simulink model "sistema_completo_despues_coloquio"  (R2023a)
settings: Solver=VariableStepAuto  StartTime=0  StopTime=15  FixedStep=1e-6  MaxStep=1e-3  RelTol=1e-3
values from neighbouring files (symbols this model uses):
  alpha_Cu = 3.9e-3    (= 0.0039)    [variables.m]
  b_a = J_eq * (2*zeta + 1) * omega_pos    [Polos_con_Jeq.m]
  b_eq = b_eq_max    [FrecuenciaNatural_Amortiguamiento.m]    (also in variables.m = 2.19444444444e-05)
  C_ts = 0.818    [variables.m]
  J_eq = J_eq_max    [FrecuenciaNatural_Amortiguamiento.m]    (also in variables.m = 4.58263888889e-05)
  k_l = m*l_cm + m_l*l_l    (= 1)    [variables.m]
  K_sa = J_eq * (2*zeta + 1) * omega_pos^2    [Polos_con_Jeq.m]
  K_sia = J_eq * omega_pos^3    [Polos_con_Jeq.m]
  L_d = 6.6e-3    (= 0.0066)    [variables.m]
  L_ls = 0.8e-3    (= 0.0008)    [variables.m]
  L_q = 5.8e-3    (= 0.0058)    [variables.m]
  lambda_m = 0.016    [variables.m]
  Pp = 3    [variables.m]
  r = 120    [esp_de_operacion.m]    (also in variables.m)
  R_ts = 146.7    [variables.m]
  T_s_ref = 20    [Polos_ceros_Rs.m]
undefined symbols (not defined in the file or in its folder): k_i, k_omega2, k_theta2, omega_n_i, omega_n_pos, omega_n_v, R_s_ref, tau, Vsl_max, zitta
libraries: SignalEditorBlockLib x5
settings Model: Creator=juanf  LastModifiedBy=Juan
settings DataIOCC: Refine=8

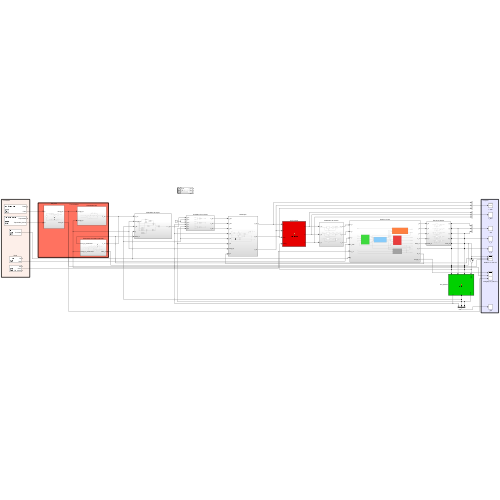
[thumbnail: Simulink's stored preview of the top-level diagram]
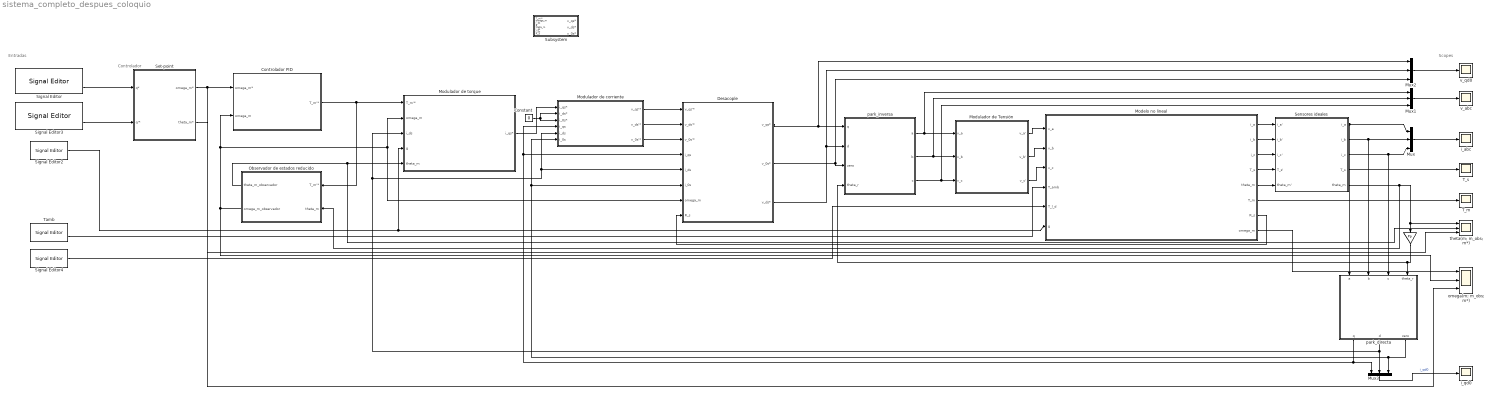
== system sistema_completo_despues_coloquio ==
  note: Controlador
  note: Scopes
  note: Entradas
  " " : Gain  Gain=Pp
  Constant : Constant  Value=0
  Controlador PID : Subsystem
  Desacople : Subsystem
  Modelo no lineal : Subsystem
  Modulador de Tensión : Subsystem
  Modulador de corriente : Subsystem
  Modulador de torque : Subsystem
  Mux{,1..3} (4 alike) : Mux  Inputs=3
  Observador de estados reducido : Subsystem
  Sensores ideales : Subsystem
  Set-point : Subsystem
  Signal Editor : SignalEditorBlockLib/Signal Editor  FileName=Consigna_Theta.mat  ActiveScenario=ConsignaTheta  ActiveSignal=Theta  IsBus=off  OutputBusObjectStr=Bus: BusObject  SampleTime=0  ZeroCross=off  OutputAfterFinalValue=Setting to zero  Unit=inherit  PreserveSignalName=on  ApplySigPropsToAllScenarios=on
  Signal Editor2 : SignalEditorBlockLib/Signal Editor  FileName=D:\Facultad\AyME\Automatica-y-maquinas-electricas-final\Matlab - Simulink\señales\g.mat  ActiveScenario=g  ActiveSignal=Constant  IsBus=off  OutputBusObjectStr=Bus: BusObject  SampleTime=0  Interpolate=off  ZeroCross=off  OutputAfterFinalValue=Setting to zero  Unit=inherit  PreserveSignalName=on  ApplySigPropsToAllScenarios=on
  Signal Editor3 : SignalEditorBlockLib/Signal Editor  FileName=D:\Facultad\AyME\Automatica-y-maquinas-electricas-final\Matlab - Simulink\señales\señal_omega_suave.mat  ActiveScenario=ConsignaOmega  ActiveSignal=Trapezoidal  IsBus=off  OutputBusObjectStr=Bus: BusObject  SampleTime=0  Interpolate=off  ZeroCross=off  OutputAfterFinalValue=Setting to zero  Unit=inherit  PreserveSignalName=on  ApplySigPropsToAllScenarios=on
  Signal Editor4 : SignalEditorBlockLib/Signal Editor  FileName=D:\Facultad\AyME\Automatica-y-maquinas-electricas-final\Matlab - Simulink\señales\Tld_15s.mat  ActiveScenario=Tld  ActiveSignal=Tld  IsBus=off  OutputBusObjectStr=Bus: BusObject  SampleTime=0  Interpolate=off  ZeroCross=off  OutputAfterFinalValue=Setting to zero  Unit=inherit  PreserveSignalName=on  ApplySigPropsToAllScenarios=on
  Subsystem : Subsystem
  T_m : Scope
  T_s : Scope
  Tamb : SignalEditorBlockLib/Signal Editor  FileName=D:\Facultad\AyME\Automatica-y-maquinas-electricas-final\Matlab - Simulink\señales\senal_Tamb.mat  ActiveScenario=T_amb  ActiveSignal=T0  IsBus=off  OutputBusObjectStr=Bus: BusObject  SampleTime=0  Interpolate=off  ZeroCross=off  OutputAfterFinalValue=Setting to zero  Unit=inherit  PreserveSignalName=on  ApplySigPropsToAllScenarios=on
  i_abc : Scope
  i_qd0 : Scope
  omega(m; m_obs; m*) : Scope  NumInputPorts=3
  park_directa : MATLAB Function  TreatAsAtomicUnit=on
  park_inversa : MATLAB Function  TreatAsAtomicUnit=on
  theta(m; m_obs; m*) : Scope  NumInputPorts=3
  v_abc : Scope
  v_qd0 : Scope
  wires:
  park_inversa/1(a) -> Mux1/1, Modulador de Tensión/1(v_a)
  park_inversa/2(b) -> Mux1/2, Modulador de Tensión/2(v_b)
  park_inversa/3(c) -> Mux1/3, Modulador de Tensión/3(v_c)
  Modulador de Tensión/1(v_a') -> Modelo no lineal/1(v_a)
  Modulador de Tensión/2(v_b') -> Modelo no lineal/2(v_b)
  Modulador de Tensión/3(v_c') -> Modelo no lineal/3(v_c)
  Modelo no lineal/1(i_a) -> Sensores ideales/1(i_a')
  Modelo no lineal/2(i_b) -> Sensores ideales/2(i_b')
  Modelo no lineal/3(i_c) -> Sensores ideales/3(i_c')
  Modelo no lineal/4(T_s) -> Sensores ideales/4(T_s')
  Modelo no lineal/5(theta_m) -> Sensores ideales/5(theta_m')
  Modelo no lineal/6(T_m) -> T_m/1
  Sensores ideales/1(i_a) -> Mux/1, park_directa/1(a)
  Sensores ideales/2(i_b) -> Mux/2, park_directa/2(b)
  Sensores ideales/3(i_c) -> Mux/3, park_directa/3(c)
  Modelo no lineal/8(omega_m) -> omega(m; m_obs; m*)/1
  Desacople/1(v_qs*) -> Mux2/1, park_inversa/1(q)
  Sensores ideales/4(T_s) -> T_s/1
  park_directa/1(q) -> Modulador de corriente/4(i_qs), Desacople/4(i_qs), Mux3/1
  park_directa/2(d) -> Mux3/2, Modulador de torque/3(i_ds), Modulador de corriente/5(i_ds), Desacople/5(i_ds)
  park_directa/3(zero) -> Mux3/3, Modulador de corriente/6(i_0s), Desacople/6(i_0s)
  Sensores ideales/5(theta_m) -> " "/1, theta(m; m_obs; m*)/1, Observador de estados reducido/2(theta_m)
  " "/1 -> park_inversa/4(theta_r), park_directa/4(theta_r)
  Mux/1 -> i_abc/1
  Mux1/1 -> v_abc/1
  Mux2/1 -> v_qd0/1
  Mux3/1 -> i_qd0/1  "i_qd0"
  Desacople/3(v_ds*) -> Mux2/2, park_inversa/2(d)
  Signal Editor2/1 -> Modulador de torque/4(g), Modelo no lineal/6(g)
  Observador de estados reducido/2(omega_m_observador) -> omega(m; m_obs; m*)/2, Controlador PID/2(omega_m), Modulador de torque/2(omega_m), Desacople/7(omega_m)
  Modulador de corriente/1(v_qs'*) -> Desacople/1(v_qs'*)
  Modulador de corriente/2(v_ds'*) -> Desacople/2(v_ds'*)
  Modulador de corriente/3(v_0s'*) -> Desacople/3(v_0s'*)
  Constant/1 -> Modulador de corriente/2(i_ds*), Modulador de corriente/3(i_0s*)
  Set-point/1(omega_m*) -> Controlador PID/1(omega_m*), omega(m; m_obs; m*)/3
  Tamb/2 -> Modelo no lineal/4(T_amb)
  Modulador de torque/1(i_qs*) -> Modulador de corriente/1(i_qs*)
  Controlador PID/1(T_m'*) -> Observador de estados reducido/1(T_m'*), Modulador de torque/1(T_m'*)
  Observador de estados reducido/1(theta_m_observador) -> theta(m; m_obs; m*)/2, Modulador de torque/5(theta_m)
  Desacople/2(v_0s*) -> park_inversa/3(zero), Mux2/3
  Modelo no lineal/7(R_s) -> Desacople/8(R_s)
  Set-point/2(theta_m*) -> theta(m; m_obs; m*)/3
  Signal Editor4/2 -> Modelo no lineal/5(T_l_d)
  Signal Editor/2 -> Set-point/1(q*)
  Signal Editor3/2 -> Set-point/2(q'*)

== system sistema_completo_despues_coloquio/Controlador PID ==
  omega_m* : Inport
  omega_m : Inport  Port=2
  Gain1 : Gain  Gain=K_sa
  Gain2 : Gain  Gain=K_sia
  Gain3 : Gain  Gain=b_a
  Integrator : Integrator
  Integrator1 : Integrator
  Sum1 : Sum  Inputs=|-+
  Sum2 : Sum  Inputs=+++
  T_m'* : Outport
  wires:
  omega_m/1 -> Sum1/1
  omega_m*/1 -> Sum1/2
  Sum1/1 -> Gain3/1, Integrator/1
  Integrator/1 -> Gain1/1, Integrator1/1
  Gain3/1 -> Sum2/3
  Gain1/1 -> Sum2/2
  Integrator1/1 -> Gain2/1
  Gain2/1 -> Sum2/1
  Sum2/1 -> T_m'*/1

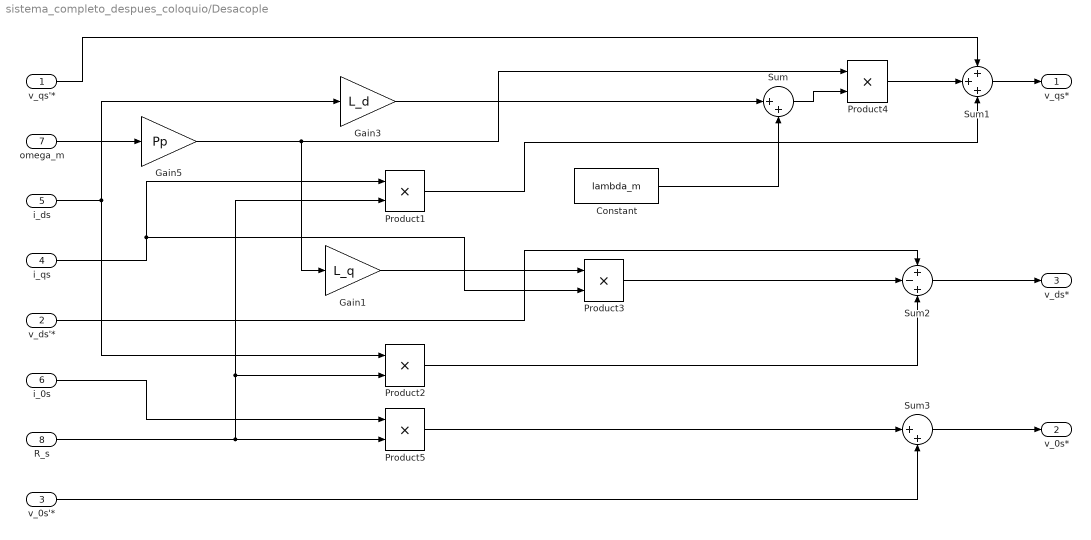
== system sistema_completo_despues_coloquio/Desacople ==
  v_qs'* : Inport
  v_ds'* : Inport  Port=2
  v_0s'* : Inport  Port=3
  i_qs : Inport  Port=4
  i_ds : Inport  Port=5
  i_0s : Inport  Port=6
  omega_m : Inport  Port=7
  R_s : Inport  Port=8
  Constant : Constant  Value=lambda_m
  Gain1 : Gain  Gain=L_q
  Gain3 : Gain  Gain=L_d
  Gain5 : Gain  Gain=Pp
  Product{1..5} (5 alike) : Product
  Sum : Sum  Inputs=|++
  Sum1 : Sum  Inputs=+++
  Sum2 : Sum  Inputs=+-+
  Sum3 : Sum  Inputs=|++
  v_qs* : Outport
  v_0s* : Outport  Port=2
  v_ds* : Outport  Port=3
  wires:
  Sum2/1 -> v_ds*/1
  Product4/1 -> Sum1/2
  R_s/1 -> Product1/2, Product2/2, Product5/2
  Gain1/1 -> Product3/1
  Product2/1 -> Sum2/3
  i_qs/1 -> Product1/1, Product3/2
  i_ds/1 -> Product2/1, Gain3/1
  v_qs'*/1 -> Sum1/1
  i_0s/1 -> Product5/1
  v_0s'*/1 -> Sum3/2
  Product3/1 -> Sum2/2
  v_ds'*/1 -> Sum2/1
  Gain5/1 -> Gain1/1, Product4/1
  omega_m/1 -> Gain5/1
  Sum/1 -> Product4/2
  Gain3/1 -> Sum/1
  Constant/1 -> Sum/2
  Sum3/1 -> v_0s*/1
  Product1/1 -> Sum1/3
  Sum1/1 -> v_qs*/1
  Product5/1 -> Sum3/1

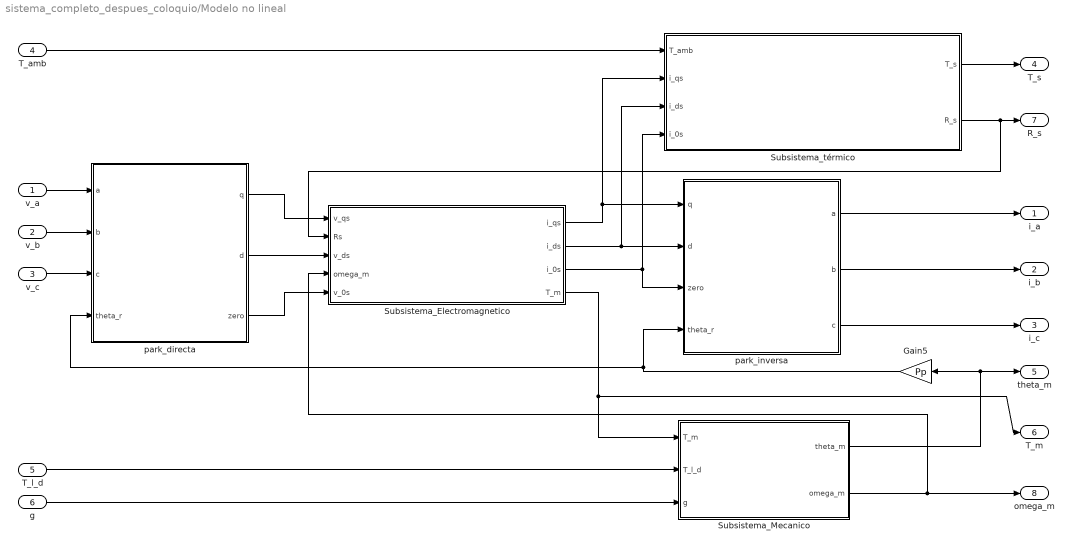
== system sistema_completo_despues_coloquio/Modelo no lineal ==
  v_a : Inport
  v_b : Inport  Port=2
  v_c : Inport  Port=3
  T_amb : Inport  Port=4
  T_l_d : Inport  Port=5
  g : Inport  Port=6
  Gain5 : Gain  Gain=Pp
  Subsistema_Electromagnetico : Subsystem
  Subsistema_Mecanico : Subsystem
  Subsistema_térmico : Subsystem
  park_directa : MATLAB Function  TreatAsAtomicUnit=on
  park_inversa : MATLAB Function  TreatAsAtomicUnit=on
  i_a : Outport
  i_b : Outport  Port=2
  i_c : Outport  Port=3
  T_s : Outport  Port=4
  theta_m : Outport  Port=5
  T_m : Outport  Port=6
  R_s : Outport  Port=7
  omega_m : Outport  Port=8
  wires:
  v_b/1 -> park_directa/2(b)
  Subsistema_Mecanico/1(theta_m) -> theta_m/1, Gain5/1
  T_l_d/1 -> Subsistema_Mecanico/2(T_l_d)
  park_directa/2(d) -> Subsistema_Electromagnetico/3(v_ds)
  Subsistema_Electromagnetico/4(T_m) -> T_m/1, Subsistema_Mecanico/1(T_m)
  T_amb/1 -> Subsistema_térmico/1(T_amb)
  Subsistema_térmico/1(T_s) -> T_s/1
  Gain5/1 -> park_directa/4(theta_r), park_inversa/4(theta_r)
  v_a/1 -> park_directa/1(a)
  Subsistema_Mecanico/2(omega_m) -> omega_m/1, Subsistema_Electromagnetico/4(omega_m)
  park_directa/1(q) -> Subsistema_Electromagnetico/1(v_qs)
  Subsistema_térmico/2(R_s) -> Subsistema_Electromagnetico/2(Rs), R_s/1
  v_c/1 -> park_directa/3(c)
  park_inversa/2(b) -> i_b/1
  Subsistema_Electromagnetico/2(i_ds) -> park_inversa/2(d), Subsistema_térmico/3(i_ds)
  park_inversa/1(a) -> i_a/1
  Subsistema_Electromagnetico/1(i_qs) -> park_inversa/1(q), Subsistema_térmico/2(i_qs)
  park_inversa/3(c) -> i_c/1
  Subsistema_Electromagnetico/3(i_0s) -> park_inversa/3(zero), Subsistema_térmico/4(i_0s)
  park_directa/3(zero) -> Subsistema_Electromagnetico/5(v_0s)
  g/1 -> Subsistema_Mecanico/3(g)

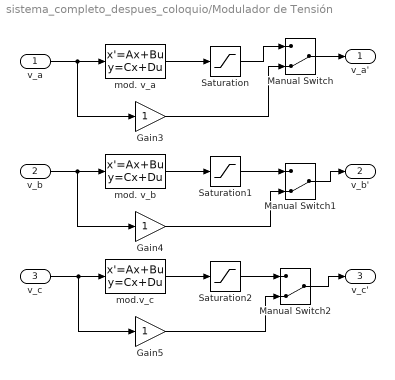
== system sistema_completo_despues_coloquio/Modulador de Tensión ==
  v_a : Inport
  v_b : Inport  Port=2
  v_c : Inport  Port=3
  Gain3 : Gain
  Gain4 : Gain
  Gain5 : Gain
  Manual Switch : ManualSwitch  CurrentSetting=0
  Manual Switch1 : ManualSwitch  CurrentSetting=0
  Manual Switch2 : ManualSwitch  CurrentSetting=0
  Saturation : Saturate  UpperLimit=Vsl_max  LowerLimit=-Vsl_max
  Saturation1 : Saturate  UpperLimit=Vsl_max  LowerLimit=-Vsl_max
  Saturation2 : Saturate  UpperLimit=Vsl_max  LowerLimit=-Vsl_max
  mod. v_a : StateSpace  A=[0 1 ; -omega_n_v^2 -2*zitta*omega_n_v]  B=[0; omega_n_v^2]  C=[1 0]  D=[0]  InitialCondition=0  AllowTunableDMatrix=on
  mod. v_b : StateSpace  A=[0 1 ; -omega_n_v^2 -2*zitta*omega_n_v]  B=[0; omega_n_v^2]  C=[1 0]  D=[0]  InitialCondition=0  AllowTunableDMatrix=on
  mod.v_c : StateSpace  A=[0 1 ; -omega_n_v^2 -2*zitta*omega_n_v]  B=[0; omega_n_v^2]  C=[1 0]  D=[0]  InitialCondition=0  AllowTunableDMatrix=on
  v_a' : Outport
  v_b' : Outport  Port=2
  v_c' : Outport  Port=3
  wires:
  v_b/1 -> mod. v_b/1, Gain4/1
  v_a/1 -> Gain3/1, mod. v_a/1
  mod. v_b/1 -> Saturation1/1
  mod.v_c/1 -> Saturation2/1
  v_c/1 -> mod.v_c/1, Gain5/1
  mod. v_a/1 -> Saturation/1
  Saturation/1 -> Manual Switch/1
  Saturation1/1 -> Manual Switch1/1
  Manual Switch/1 -> v_a'/1
  Gain3/1 -> Manual Switch/2
  Gain4/1 -> Manual Switch1/2
  Manual Switch1/1 -> v_b'/1
  Saturation2/1 -> Manual Switch2/1
  Manual Switch2/1 -> v_c'/1
  Gain5/1 -> Manual Switch2/2

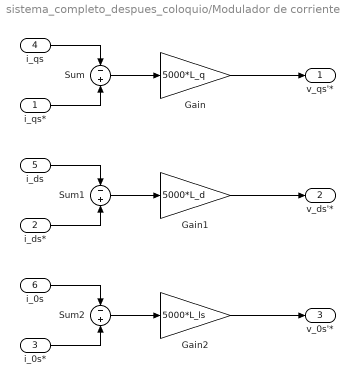
== system sistema_completo_despues_coloquio/Modulador de corriente ==
  i_qs* : Inport
  i_ds* : Inport  Port=2
  i_0s* : Inport  Port=3
  i_qs : Inport  Port=4
  i_ds : Inport  Port=5
  i_0s : Inport  Port=6
  Gain : Gain  Gain=5000*L_q
  Gain1 : Gain  Gain=5000*L_d
  Gain2 : Gain  Gain=5000*L_ls
  Sum : Sum  Inputs=-|+
  Sum1 : Sum  Inputs=-|+
  Sum2 : Sum  Inputs=-|+
  v_qs'* : Outport
  v_ds'* : Outport  Port=2
  v_0s'* : Outport  Port=3
  wires:
  i_qs/1 -> Sum/1
  i_qs*/1 -> Sum/2
  Sum/1 -> Gain/1
  Gain/1 -> v_qs'*/1
  i_ds/1 -> Sum1/1
  i_ds*/1 -> Sum1/2
  Sum1/1 -> Gain1/1
  Gain1/1 -> v_ds'*/1
  i_0s/1 -> Sum2/1
  i_0s*/1 -> Sum2/2
  Sum2/1 -> Gain2/1
  Gain2/1 -> v_0s'*/1

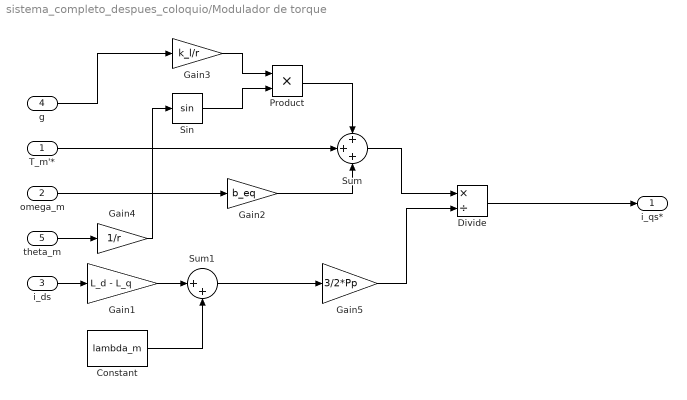
== system sistema_completo_despues_coloquio/Modulador de torque ==
  T_m'* : Inport
  omega_m : Inport  Port=2
  i_ds : Inport  Port=3
  g : Inport  Port=4
  theta_m : Inport  Port=5
  Constant : Constant  Value=lambda_m
  Divide : Product  Inputs=*/
  Gain1 : Gain  Gain=L_d - L_q
  Gain2 : Gain  Gain=b_eq
  Gain3 : Gain  Gain=k_l/r
  Gain4 : Gain  Gain=1/r
  Gain5 : Gain  Gain=3/2*Pp
  Product : Product
  Sin : Trigonometry
  Sum : Sum  Inputs=+++
  Sum1 : Sum  Inputs=|++
  i_qs* : Outport
  wires:
  Sum1/1 -> Gain5/1
  omega_m/1 -> Gain2/1
  T_m'*/1 -> Sum/2
  Gain2/1 -> Sum/3
  i_ds/1 -> Gain1/1
  Gain1/1 -> Sum1/1
  Constant/1 -> Sum1/2
  g/1 -> Gain3/1
  theta_m/1 -> Gain4/1
  Gain4/1 -> Sin/1
  Gain3/1 -> Product/1
  Sin/1 -> Product/2
  Product/1 -> Sum/1
  Sum/1 -> Divide/1
  Gain5/1 -> Divide/2
  Divide/1 -> i_qs*/1

== system sistema_completo_despues_coloquio/Observador de estados reducido ==
  T_m'* : Inport
  theta_m : Inport  Port=2
  Gain : Gain  Gain=k_omega2
  Gain1 : Gain  Gain=k_theta2
  Gain2 : Gain  Gain=1/J_eq
  Gain3 : Gain  Gain=k_i
  Integrator : Integrator
  Integrator1 : Integrator
  Integrator2 : Integrator
  Sum : Sum  Inputs=|+-
  Sum2 : Sum  Inputs=+++
  Sum3 : Sum  Inputs=|++
  theta_m_observador : Outport
  omega_m_observador : Outport  Port=2
  wires:
  theta_m/1 -> Sum/1
  Sum2/1 -> Integrator1/1
  T_m'*/1 -> Gain2/1
  Sum/1 -> Gain/1, Gain1/1, Integrator2/1
  Sum3/1 -> Integrator/1, omega_m_observador/1
  Integrator/1 -> Sum/2, theta_m_observador/1
  Integrator1/1 -> Sum3/1
  Gain1/1 -> Sum3/2
  Gain2/1 -> Sum2/2
  Gain/1 -> Sum2/3
  Integrator2/1 -> Gain3/1
  Gain3/1 -> Sum2/1

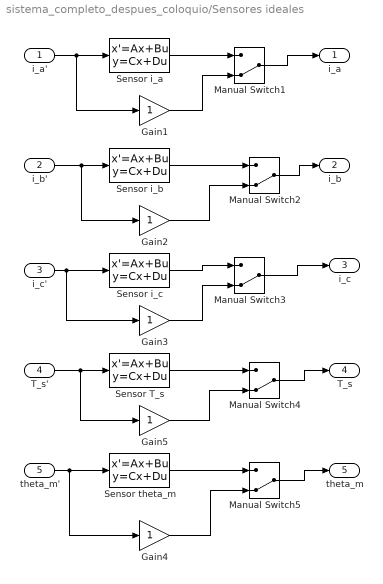
== system sistema_completo_despues_coloquio/Sensores ideales ==
  i_a' : Inport
  i_b' : Inport  Port=2
  i_c' : Inport  Port=3
  T_s' : Inport  Port=4
  theta_m' : Inport  Port=5
  Gain{1..5} (5 alike) : Gain
  Manual Switch{1..5} (5 alike) : ManualSwitch  CurrentSetting=0
  Sensor T_s : StateSpace  A=[-1/tau]  B=[1/tau]  C=[1]  D=[0]  InitialCondition=40  AllowTunableDMatrix=on
  Sensor i_a : StateSpace  A=[0 1 ; -omega_n_i^2 -2*zitta*omega_n_i]  B=[0; omega_n_i^2]  C=[1 0]  D=[0]  InitialCondition=0  AllowTunableDMatrix=on
  Sensor i_b : StateSpace  A=[0 1 ; -omega_n_i^2 -2*zitta*omega_n_i]  B=[0; omega_n_i^2]  C=[1 0]  D=[0]  InitialCondition=0  AllowTunableDMatrix=on
  Sensor i_c : StateSpace  A=[0 1 ; -omega_n_i^2 -2*zitta*omega_n_i]  B=[0; omega_n_i^2]  C=[1 0]  D=[0]  InitialCondition=0  AllowTunableDMatrix=on
  Sensor theta_m : StateSpace  A=[0 1 ; -omega_n_pos^2 -2*zitta*omega_n_pos]  B=[0; omega_n_pos^2]  C=[1 0]  D=[0]  InitialCondition=0  AllowTunableDMatrix=on
  i_a : Outport
  i_b : Outport  Port=2
  i_c : Outport  Port=3
  T_s : Outport  Port=4
  theta_m : Outport  Port=5
  wires:
  i_a'/1 -> Gain1/1, Sensor i_a/1
  i_b'/1 -> Gain2/1, Sensor i_b/1
  i_c'/1 -> Gain3/1, Sensor i_c/1
  T_s'/1 -> Gain5/1, Sensor T_s/1
  theta_m'/1 -> Gain4/1, Sensor theta_m/1
  Sensor i_a/1 -> Manual Switch1/1
  Sensor i_b/1 -> Manual Switch2/1
  Sensor T_s/1 -> Manual Switch4/1
  Sensor theta_m/1 -> Manual Switch5/1
  Manual Switch1/1 -> i_a/1
  Gain1/1 -> Manual Switch1/2
  Gain2/1 -> Manual Switch2/2
  Manual Switch2/1 -> i_b/1
  Sensor i_c/1 -> Manual Switch3/1
  Gain3/1 -> Manual Switch3/2
  Manual Switch3/1 -> i_c/1
  Gain5/1 -> Manual Switch4/2
  Manual Switch4/1 -> T_s/1
  Gain4/1 -> Manual Switch5/2
  Manual Switch5/1 -> theta_m/1

== system sistema_completo_despues_coloquio/Set-point ==
  q* : Inport
  q'* : Inport  Port=2
  Derivative : Derivative
  Gain : Gain  Gain=r
  Gain1 : Gain  Gain=r
  Integrator : Integrator
  Manual Switch : ManualSwitch  CurrentSetting=0
  Manual Switch1 : ManualSwitch
  omega_m* : Outport
  theta_m* : Outport  Port=2
  wires:
  q*/1 -> Gain/1
  Manual Switch/1 -> theta_m*/1
  Gain/1 -> Manual Switch/1, Derivative/1
  Gain1/1 -> Integrator/1, Manual Switch1/1
  Integrator/1 -> Manual Switch/2
  Derivative/1 -> Manual Switch1/2
  q'*/1 -> Gain1/1
  Manual Switch1/1 -> omega_m*/1

== system sistema_completo_despues_coloquio/Subsystem ==
  T_m'* : Inport
  omega_m : Inport  Port=2
  i_ds : Inport  Port=3
  g : Inport  Port=4
  theta_m : Inport  Port=5
  i_qs : Inport  Port=6
  i_0s : Inport  Port=7
  R_s : Inport  Port=8
  Constant : Constant  Value=0
  Desacople : Subsystem
  Lazo de corriente : Subsystem
  Lazo de torque : Subsystem
  v_qs* : Outport
  v_ds* : Outport  Port=2
  v_0s* : Outport  Port=3
  wires:
  Lazo de torque/1(i_qs*) -> Lazo de corriente/1(i_qs*)
  Lazo de corriente/1(v_qs'*) -> Desacople/1(v_qs'*)
  Lazo de corriente/2(v_ds'*) -> Desacople/2(v_ds'*)
  Lazo de corriente/3(v_0s'*) -> Desacople/3(v_0s'*)
  i_qs/1 -> Lazo de corriente/4(i_qs), Desacople/4(i_qs)
  T_m'*/1 -> Lazo de torque/1(T_m'*)
  omega_m/1 -> Desacople/7(omega_m), Lazo de torque/2(omega_m)
  i_ds/1 -> Lazo de corriente/5(i_ds), Desacople/5(i_ds), Lazo de torque/3(i_ds)
  g/1 -> Lazo de torque/4(g)
  theta_m/1 -> Lazo de torque/5(theta_m)
  i_0s/1 -> Lazo de corriente/6(i_0s), Desacople/6(i_0s)
  Constant/1 -> Lazo de corriente/3(i_0s*), Lazo de corriente/2(i_ds*)
  R_s/1 -> Desacople/8(R_s)
  Desacople/1(v_qs*) -> v_qs*/1
  Desacople/2(v_ds*) -> v_ds*/1
  Desacople/3(v_0s*) -> v_0s*/1

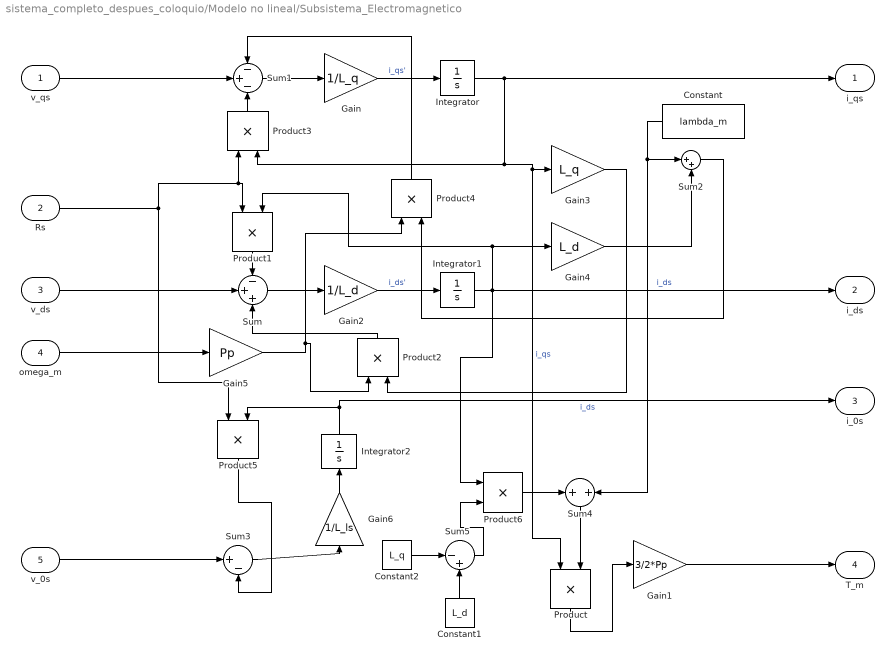
== system sistema_completo_despues_coloquio/Modelo no lineal/Subsistema_Electromagnetico ==
  v_qs : Inport
  Rs : Inport  Port=2
  v_ds : Inport  Port=3
  omega_m : Inport  Port=4
  v_0s : Inport  Port=5
  Constant : Constant  Value=lambda_m
  Constant1 : Constant  Value=L_d
  Constant2 : Constant  Value=L_q
  Gain : Gain  Gain=1/L_q
  Gain1 : Gain  Gain=3/2*Pp
  Gain2 : Gain  Gain=1/L_d
  Gain3 : Gain  Gain=L_q
  Gain4 : Gain  Gain=L_d
  Gain5 : Gain  Gain=Pp
  Gain6 : Gain  Gain=1/L_ls
  Integrator : Integrator
  Integrator1 : Integrator
  Integrator2 : Integrator
  Product{,1..6} (7 alike) : Product
  Sum : Sum  Inputs=-++
  Sum1 : Sum  Inputs=-+-
  Sum2 : Sum  Inputs=|++
  Sum3 : Sum  Inputs=|+-
  Sum4 : Sum
  Sum5 : Sum  Inputs=|-+
  i_qs : Outport
  i_ds : Outport  Port=2
  i_0s : Outport  Port=3
  T_m : Outport  Port=4
  wires:
  Gain1/1 -> T_m/1
  Product/1 -> Gain1/1
  v_qs/1 -> Sum1/2
  Sum1/1 -> Gain/1
  Gain/1 -> Integrator/1  "i_qs'"
  Integrator/1 -> Product/1, Gain3/1, Product3/2, i_qs/1  "i_qs"
  Product3/1 -> Sum1/3
  Rs/1 -> Product3/1, Product1/1, Product5/1
  Product4/1 -> Sum1/1
  Product1/1 -> Sum/1
  v_ds/1 -> Sum/2
  Sum/1 -> Gain2/1
  Gain2/1 -> Integrator1/1  "i_ds'"
  Integrator1/1 -> i_ds/1, Product6/1, Gain4/1, Product1/2  "i_ds"
  Constant/1 -> Sum4/2, Sum2/1
  Sum2/1 -> Product4/2
  omega_m/1 -> Gain5/1
  Gain5/1 -> Product2/1, Product4/1
  Product2/1 -> Sum/3
  Gain4/1 -> Sum2/2
  Gain3/1 -> Product2/2
  v_0s/1 -> Sum3/1
  Product5/1 -> Sum3/2
  Sum3/1 -> Gain6/1
  Gain6/1 -> Integrator2/1
  Integrator2/1 -> Product5/2, i_0s/1  "i_ds"
  Constant1/1 -> Sum5/2
  Constant2/1 -> Sum5/1
  Product6/1 -> Sum4/1
  Sum5/1 -> Product6/2
  Sum4/1 -> Product/2

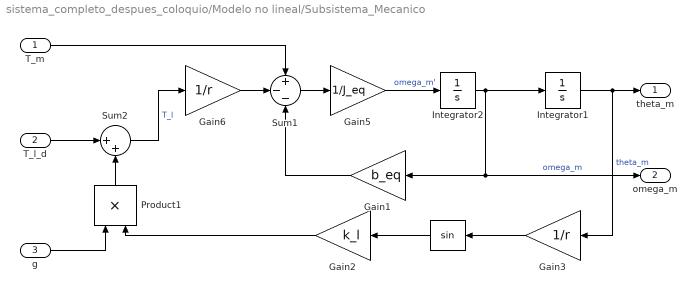
== system sistema_completo_despues_coloquio/Modelo no lineal/Subsistema_Mecanico ==
  T_m : Inport
  T_l_d : Inport  Port=2
  g : Inport  Port=3
  " " : Trigonometry
  Gain1 : Gain  Gain=b_eq
  Gain2 : Gain  Gain=k_l
  Gain3 : Gain  Gain=1/r
  Gain5 : Gain  Gain=1/J_eq
  Gain6 : Gain  Gain=1/r
  Integrator1 : Integrator
  Integrator2 : Integrator
  Product1 : Product
  Sum1 : Sum  Inputs=+--
  Sum2 : Sum  Inputs=|++
  theta_m : Outport
  omega_m : Outport  Port=2
  wires:
  Product1/1 -> Sum2/2
  T_l_d/1 -> Sum2/1
  Integrator1/1 -> theta_m/1, Gain3/1  "theta_m"
  Gain3/1 -> " "/1
  " "/1 -> Gain2/1
  Gain1/1 -> Sum1/3
  Sum1/1 -> Gain5/1
  Sum2/1 -> Gain6/1  "T_l"
  Gain6/1 -> Sum1/2
  Integrator2/1 -> Integrator1/1, Gain1/1, omega_m/1  "omega_m"
  Gain5/1 -> Integrator2/1  "omega_m'"
  Gain2/1 -> Product1/2
  T_m/1 -> Sum1/1
  g/1 -> Product1/1

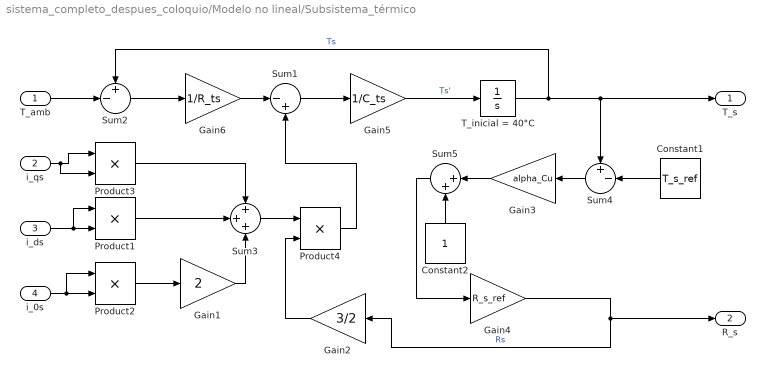
== system sistema_completo_despues_coloquio/Modelo no lineal/Subsistema_térmico ==
  T_amb : Inport
  i_qs : Inport  Port=2
  i_ds : Inport  Port=3
  i_0s : Inport  Port=4
  Constant1 : Constant  Value=T_s_ref
  Constant2 : Constant
  Gain1 : Gain  Gain=2
  Gain2 : Gain  Gain=3/2
  Gain3 : Gain  Gain=alpha_Cu
  Gain4 : Gain  Gain=R_s_ref
  Gain5 : Gain  Gain=1/C_ts
  Gain6 : Gain  Gain=1/R_ts
  Product{1..4} (4 alike) : Product
  Sum1 : Sum  Inputs=|-+
  Sum2 : Sum  Inputs=+-|
  Sum3 : Sum  Inputs=+++
  Sum4 : Sum  Inputs=+-|
  Sum5 : Sum  Inputs=|++
  T_inicial = 40°C : Integrator  InitialCondition=40
  T_s : Outport
  R_s : Outport  Port=2
  wires:
  Gain5/1 -> T_inicial = 40°C/1  "Ts'"
  Sum1/1 -> Gain5/1
  Sum2/1 -> Gain6/1
  T_amb/1 -> Sum2/2
  T_inicial = 40°C/1 -> Sum4/1, T_s/1, Sum2/1  "Ts"
  i_qs/1 -> Product3/2, Product3/1
  i_0s/1 -> Product2/1, Product2/2
  Product2/1 -> Gain1/1
  Gain1/1 -> Sum3/3
  Product1/1 -> Sum3/2
  Product3/1 -> Sum3/1
  Sum3/1 -> Product4/1
  Gain2/1 -> Product4/2
  Gain6/1 -> Sum1/1
  Product4/1 -> Sum1/2
  Constant1/1 -> Sum4/2
  Sum4/1 -> Gain3/1
  Constant2/1 -> Sum5/2
  Sum5/1 -> Gain4/1
  Gain4/1 -> Gain2/1, R_s/1  "Rs"
  Gain3/1 -> Sum5/1
  i_ds/1 -> Product1/2, Product1/1

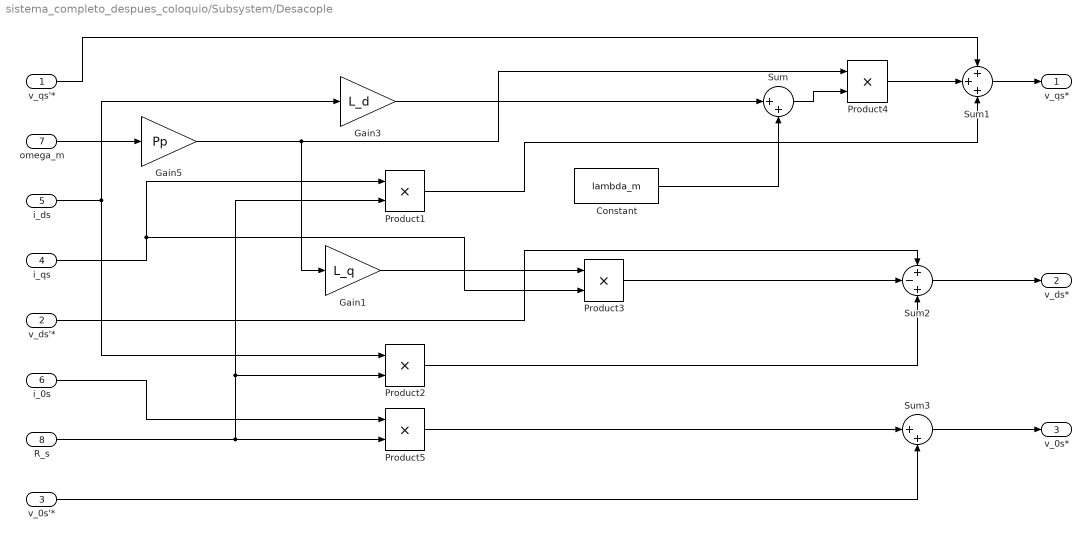
== system sistema_completo_despues_coloquio/Subsystem/Desacople ==
  v_qs'* : Inport
  v_ds'* : Inport  Port=2
  v_0s'* : Inport  Port=3
  i_qs : Inport  Port=4
  i_ds : Inport  Port=5
  i_0s : Inport  Port=6
  omega_m : Inport  Port=7
  R_s : Inport  Port=8
  Constant : Constant  Value=lambda_m
  Gain1 : Gain  Gain=L_q
  Gain3 : Gain  Gain=L_d
  Gain5 : Gain  Gain=Pp
  Product{1..5} (5 alike) : Product
  Sum : Sum  Inputs=|++
  Sum1 : Sum  Inputs=+++
  Sum2 : Sum  Inputs=+-+
  Sum3 : Sum  Inputs=|++
  v_qs* : Outport
  v_ds* : Outport  Port=2
  v_0s* : Outport  Port=3
  wires:
  Sum2/1 -> v_ds*/1
  Product4/1 -> Sum1/2
  R_s/1 -> Product1/2, Product2/2, Product5/2
  Gain1/1 -> Product3/1
  Product2/1 -> Sum2/3
  i_qs/1 -> Product1/1, Product3/2
  i_ds/1 -> Product2/1, Gain3/1
  v_qs'*/1 -> Sum1/1
  i_0s/1 -> Product5/1
  v_0s'*/1 -> Sum3/2
  Product3/1 -> Sum2/2
  v_ds'*/1 -> Sum2/1
  Gain5/1 -> Gain1/1, Product4/1
  omega_m/1 -> Gain5/1
  Sum/1 -> Product4/2
  Gain3/1 -> Sum/1
  Constant/1 -> Sum/2
  Sum3/1 -> v_0s*/1
  Product1/1 -> Sum1/3
  Sum1/1 -> v_qs*/1
  Product5/1 -> Sum3/1

== system sistema_completo_despues_coloquio/Subsystem/Lazo de corriente ==
  i_qs* : Inport
  i_ds* : Inport  Port=2
  i_0s* : Inport  Port=3
  i_qs : Inport  Port=4
  i_ds : Inport  Port=5
  i_0s : Inport  Port=6
  Gain : Gain  Gain=5000*L_q
  Gain1 : Gain  Gain=5000*L_d
  Gain2 : Gain  Gain=5000*L_ls
  Sum : Sum  Inputs=-|+
  Sum1 : Sum  Inputs=-|+
  Sum2 : Sum  Inputs=-|+
  v_qs'* : Outport
  v_ds'* : Outport  Port=2
  v_0s'* : Outport  Port=3
  wires:
  i_qs/1 -> Sum/1
  i_qs*/1 -> Sum/2
  Sum/1 -> Gain/1
  Gain/1 -> v_qs'*/1
  i_ds/1 -> Sum1/1
  i_ds*/1 -> Sum1/2
  Sum1/1 -> Gain1/1
  Gain1/1 -> v_ds'*/1
  i_0s/1 -> Sum2/1
  i_0s*/1 -> Sum2/2
  Sum2/1 -> Gain2/1
  Gain2/1 -> v_0s'*/1

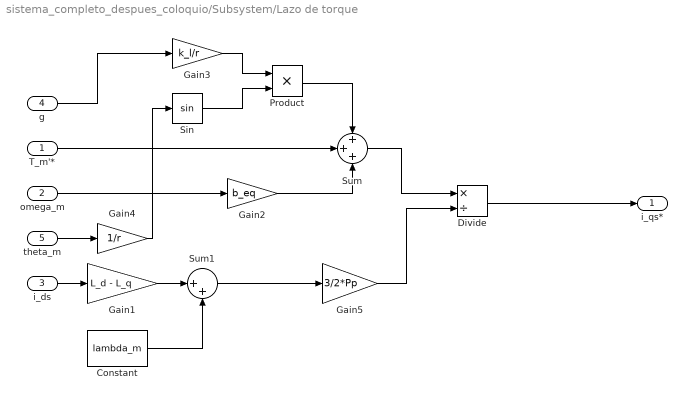
== system sistema_completo_despues_coloquio/Subsystem/Lazo de torque ==
  T_m'* : Inport
  omega_m : Inport  Port=2
  i_ds : Inport  Port=3
  g : Inport  Port=4
  theta_m : Inport  Port=5
  Constant : Constant  Value=lambda_m
  Divide : Product  Inputs=*/
  Gain1 : Gain  Gain=L_d - L_q
  Gain2 : Gain  Gain=b_eq
  Gain3 : Gain  Gain=k_l/r
  Gain4 : Gain  Gain=1/r
  Gain5 : Gain  Gain=3/2*Pp
  Product : Product
  Sin : Trigonometry
  Sum : Sum  Inputs=+++
  Sum1 : Sum  Inputs=|++
  i_qs* : Outport
  wires:
  Sum1/1 -> Gain5/1
  omega_m/1 -> Gain2/1
  T_m'*/1 -> Sum/2
  Gain2/1 -> Sum/3
  i_ds/1 -> Gain1/1
  Gain1/1 -> Sum1/1
  Constant/1 -> Sum1/2
  g/1 -> Gain3/1
  theta_m/1 -> Gain4/1
  Gain4/1 -> Sin/1
  Gain3/1 -> Product/1
  Sin/1 -> Product/2
  Product/1 -> Sum/1
  Sum/1 -> Divide/1
  Gain5/1 -> Divide/2
  Divide/1 -> i_qs*/1

== matlab function sistema_completo_despues_coloquio/park_inversa ==
  data: q input; a output; d input; zero input; theta_r input; b output; c output
function [a, b, c] = park_inversa(q, d, zero, theta_r)
% qd0 → abc (transformacion inversa)
% Entradas: q, d, zero (coordenadas qd0), theta_r (ángulo eléctrico)
% Salidas: a, b, c (señales de fase)
    
    T_inv = [cos(theta_r),               sin(theta_r),              1;
             cos(theta_r - 2*pi/3),      sin(theta_r - 2*pi/3),     1;
             cos(theta_r + 2*pi/3),      sin(theta_r + 2*pi/3),     1];
    
    abc = T_inv * [q; d; zero];

    a = abc(1);
    b = abc(2);
    c = abc(3);
end

== matlab function sistema_completo_despues_coloquio/park_directa ==
  data: a input; q output; b input; c input; theta_r input; d output; zero output
function [q, d, zero] = park_directa(a, b, c, theta_r)
% Transformacion abc → qd0
% a, b y c son señales de fase y theta_r es el angulo ELECTRICO (no mecanico) del rotor)
% Salidas: q, d, zero, que son las coordenadas virtuales qd0
    
    T = (2/3) * [cos(theta_r),           cos(theta_r - 2*pi/3),      cos(theta_r + 2*pi/3);
                 sin(theta_r),           sin(theta_r - 2*pi/3),      sin(theta_r + 2*pi/3);
                 1/2,                    1/2,                         1/2];
    
    qd0 = T * [a; b; c];
    
% asignar salidas
    q = qd0(1);
    d = qd0(2);
    zero = qd0(3);
end

== matlab function sistema_completo_despues_coloquio/Modelo no lineal/park_directa ==
  data: a input; q output; b input; c input; theta_r input; d output; zero output
function [q, d, zero] = park_directa(a, b, c, theta_r)
% Transformacion abc → qd0
% a, b y c son señales de fase y theta_r es el angulo ELECTRICO (no mecanico) del rotor)
% Salidas: q, d, zero, que son las coordenadas virtuales qd0
    
    T = (2/3) * [cos(theta_r),           cos(theta_r - 2*pi/3),      cos(theta_r + 2*pi/3);
                 sin(theta_r),           sin(theta_r - 2*pi/3),      sin(theta_r + 2*pi/3);
                 1/2,                    1/2,                         1/2];
    
    qd0 = T * [a; b; c];
    
% asignar salidas
    q = qd0(1);
    d = qd0(2);
    zero = qd0(3);
end

== matlab function sistema_completo_despues_coloquio/Modelo no lineal/park_inversa ==
  data: q input; a output; d input; zero input; theta_r input; b output; c output
function [a, b, c] = park_inversa(q, d, zero, theta_r)
% qd0 → abc (transformacion inversa)
% Entradas: q, d, zero (coordenadas qd0), theta_r (ángulo eléctrico)
% Salidas: a, b, c (señales de fase)
    
    T_inv = [cos(theta_r),               sin(theta_r),              1;
             cos(theta_r - 2*pi/3),      sin(theta_r - 2*pi/3),     1;
             cos(theta_r + 2*pi/3),      sin(theta_r + 2*pi/3),     1];
    
    abc = T_inv * [q; d; zero];

    a = abc(1);
    b = abc(2);
    c = abc(3);
end
